simulink model "proiect_date_modificateV2"  (R2022b)
settings: Solver=VariableStepAuto  StartTime=0.0  StopTime=2500  RelTol=1e-3
values from neighbouring files (symbols this model uses):
  C = 9    [Coeficienti_Pompa.m]    (also in Coeficienti_Pompa_Modificati.m = 5.75; Coeficienti_Pompa_ModificatiV2.m = 7.55)
  k = 0.035    [Coeficienti_Pompa.m]    (also in Coeficienti_Pompa_Modificati.m = 0.025; Coeficienti_Pompa_ModificatiV2.m = 0.037)
  k1 = 0.624    [Coeficienti_Pompa.m]    (also in Coeficienti_Pompa_Modificati.m; Coeficienti_Pompa_ModificatiV2.m)
  k11 = k2^2 + 4* (k - k3) * k1    (= 0.0890826)    [Coeficienti_Pompa.m]    (also in Coeficienti_Pompa_Modificati.m = 0.0641226; Coeficienti_Pompa_ModificatiV2.m = 0.0940746)
  k12 = 8* (k - k3) * h    (= 0.2848)    [Coeficienti_Pompa.m]    (also in Coeficienti_Pompa_Modificati.m = 0.2048; Coeficienti_Pompa_ModificatiV2.m = 0.3008)
  k13 = 2* (k - k3)    (= 0.0712)    [Coeficienti_Pompa.m]    (also in Coeficienti_Pompa_Modificati.m = 0.0512; Coeficienti_Pompa_ModificatiV2.m = 0.0752)
  k2 = -0.015    [Coeficienti_Pompa.m]    (also in Coeficienti_Pompa_Modificati.m; Coeficienti_Pompa_ModificatiV2.m)
  k3 = -0.0006    [Coeficienti_Pompa.m]    (also in Coeficienti_Pompa_Modificati.m; Coeficienti_Pompa_ModificatiV2.m)
  kcompensare = (deltah/deltaq)/(deltah/deltau)    (= 0.1)    [Coeficienti_Pompa.m]    (also in Coeficienti_Pompa_Modificati.m; Coeficienti_Pompa_ModificatiV2.m)
  keta = 8e-5    (= 8e-05)    [Coeficienti_Pompa.m]    (also in Coeficienti_Pompa_Modificati.m; Coeficienti_Pompa_ModificatiV2.m)
libraries: slpidlib x7
(part 2 of 2)

== system proiect_date_modificateV2/FF/sistem_feedforward/Pompa  ==
  kn : Inport
  h : Inport  Port=2
  Gain : Gain  Gain=k2
  Gain1 : Gain  Gain=k11
  Gain2 : Gain  Gain=k12
  Gain3 : Gain  Gain=1/k13
  Product : Product
  Sqrt : Sqrt
  Subtract1 : Sum  Inputs=+-
  substract : Sum
  q : Outport
  wires:
  Gain3/1 -> q/1
  Subtract1/1 -> Sqrt/1
  Gain/1 -> substract/1
  h/1 -> Gain2/1
  Product/1 -> Gain1/1
  Gain1/1 -> Subtract1/1
  Gain2/1 -> Subtract1/2
  Sqrt/1 -> substract/2
  kn/1 -> Gain/1, Product/2, Product/1
  substract/1 -> Gain3/1

== system proiect_date_modificateV2/FF/sistem_feedforward/Randament ==
  q : Inport
  um : Inport  Port=2
  Gain : Gain  Gain=keta
  Product : Product
  eta : Outport
  wires:
  Product/1 -> eta/1
  um/1 -> Gain/1
  Gain/1 -> Product/2
  q/1 -> Product/1

== system proiect_date_modificateV2/FF/sistem_feedforward/rezervor_feedforward ==
  q1 : Inport
  Add : Sum
  C : Constant  Value=C
  Gain : Gain  Gain=1/332.5
  Integrator : Integrator  InitialCondition=10.5
  Product : Product
  Product1 : Product
  Scope : Scope
  Sqrt : Sqrt  IntermediateResultsDataTypeStr=double
  Step : Step  Time=500  After=2  SampleTime=0
  Sum : Sum  Inputs=|+-
  h1 : Outport
  perturabtie : Outport  Port=2
  wires:
  Product1/1 -> perturabtie/1
  Integrator/1 -> h1/1, Sqrt/1
  C/1 -> Add/2
  Product/1 -> Scope/1, Sum/2
  Add/1 -> Product/2
  Sqrt/1 -> Product1/1, Product/1
  Step/1 -> Product1/2, Add/1
  Sum/1 -> Gain/1
  Gain/1 -> Integrator/1
  q1/1 -> Sum/1
